simulink model "Simulink_X_Com_Restricao"  (Simulink 8.2)
settings: Solver=ode4  SolverMode=SingleTasking  StartTime=0.0  StopTime=100  FixedStep=0.01  RelTol=1e-3
InitFcn:
  | Main_Simulink_X_Com_Restricao;
values from neighbouring files (symbols this model uses):
  A1 = [ 0.1   10 ... (first row only)    [MatrizesEspacoEstados.m]
  B1 = [0 ... (first row only)    [MatrizesEspacoEstados.m]
  C = eye(theta)    [MatrizesEspacoEstados.m]
  D = 0*C(:,theta)    [MatrizesEspacoEstados.m]
  xk0 = [3; 5]    [xk_0.m]
undefined symbols (not defined in the file): A, B, rho, Umax
settings Model: Creator=Kawakami  LastModifiedBy=Eduardo
settings DataIOCC: LimitDataPoints=off  SaveOutput=off  SaveTime=off  TimeSaveName=t  SignalLoggingName=sigsOut
settings OptimizationCC: BooleanDataType=off
settings DebuggingCC: SaveWithParameterizedLinksMsg=none  SignalResolutionControl=TryResolveAllWithWarning  SolverPrmCheckMsg=none  MultiTaskDSMMsg=warning  MultiTaskCondExecSysMsg=none
settings HardwareCC: TargetUnknown=on
settings RTWCC: IncludeERTFirstTime=on

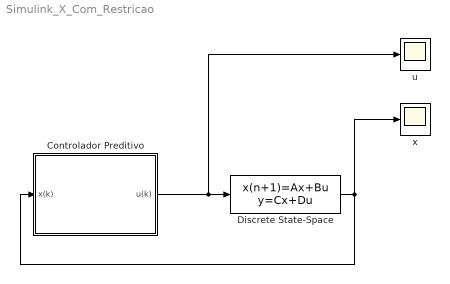
== system Simulink_X_Com_Restricao ==
  "Controlador Preditivo  " : Subsystem  mask{A=A, B=B, H=Umax, rho=rho, T=1}
      mask prompts: A "Matriz Agregada A"; B "Matriz Agregada B"; H "Matriz H"; rho "Peso do Gamma"; T "T (passo da simulação)"
  Discrete State-Space : DiscreteStateSpace  A=A1  B=B1  C=C  D=D  X0=xk0
  u : Scope
      settings: TimeRange=10  YMin=-2  YMax=0.5
  x : Scope
      settings: YMin=-1.25  YMax=2.25
  wires:
  "Controlador Preditivo  "/1(u(k)) -> u/1, Discrete State-Space/1
  Discrete State-Space/1 -> x/1, "Controlador Preditivo  "/1(x(k))

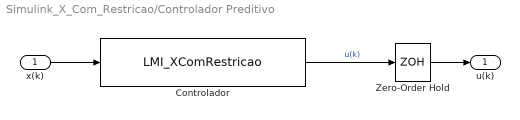
== system Simulink_X_Com_Restricao/Controlador Preditivo   ==
  x(k) : Inport
  Controlador : S-Function  FunctionName=LMI_XComRestricao  Parameters=A, B, Umax, rho, T  EnableBusSupport=off
  Zero-Order Hold : ZeroOrderHold  SampleTime=T
  u(k) : Outport
  wires:
  Zero-Order Hold/1 -> u(k)/1
  x(k)/1 -> Controlador/1
  Controlador/1 -> Zero-Order Hold/1  "u(k)"
